simulink model "SwitchActionSubsystem"  (R2021a)
settings: Solver=VariableStepAuto  StartTime=0.0  StopTime=10.0  RelTol=1e-3
settings Model: Creator=lenovo  LastModifiedBy=lenovo

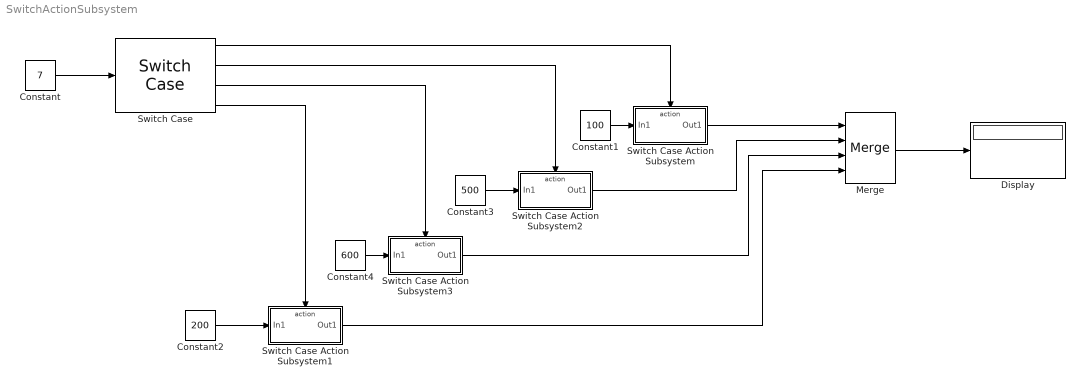
== system SwitchActionSubsystem ==
  Constant : Constant  Value=7
  Constant1 : Constant  Value=100
  Constant2 : Constant  Value=200
  Constant3 : Constant  Value=500
  Constant4 : Constant  Value=600
  Display : Display
  Merge : Merge  Inputs=4
  Switch Case : SwitchCase  CaseConditions={1,2,[4 5]}
  Switch Case Action Subsystem : Subsystem  TreatAsAtomicUnit=on
  Switch Case Action Subsystem1 : Subsystem  TreatAsAtomicUnit=on
  Switch Case Action Subsystem2 : Subsystem  TreatAsAtomicUnit=on
  Switch Case Action Subsystem3 : Subsystem  TreatAsAtomicUnit=on
  wires:
  Constant/1 -> Switch Case/1
  Switch Case/1 -> Switch Case Action Subsystem/Action
  Constant1/1 -> Switch Case Action Subsystem/1(In1)
  Constant2/1 -> Switch Case Action Subsystem1/1(In1)
  Constant3/1 -> Switch Case Action Subsystem2/1(In1)
  Switch Case/2 -> Switch Case Action Subsystem2/Action
  Switch Case/3 -> Switch Case Action Subsystem3/Action
  Constant4/1 -> Switch Case Action Subsystem3/1(In1)
  Switch Case/4 -> Switch Case Action Subsystem1/Action
  Switch Case Action Subsystem/1(Out1) -> Merge/1
  Switch Case Action Subsystem2/1(Out1) -> Merge/2
  Switch Case Action Subsystem3/1(Out1) -> Merge/3
  Switch Case Action Subsystem1/1(Out1) -> Merge/4
  Merge/1 -> Display/1

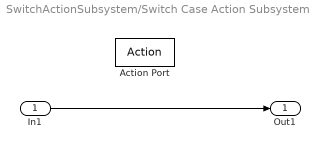
== system SwitchActionSubsystem/Switch Case Action Subsystem ==
  In1 : Inport
  Action Port : ActionPort  ActionPortLabel=case [ 1 ]:
  Out1 : Outport
  wires:
  In1/1 -> Out1/1

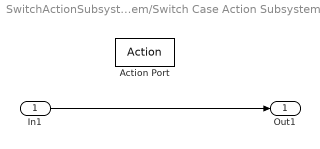
== system SwitchActionSubsystem/Switch Case Action Subsystem1 ==
  In1 : Inport
  Action Port : ActionPort  ActionPortLabel=default:
  Out1 : Outport
  wires:
  In1/1 -> Out1/1

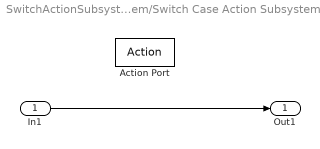
== system SwitchActionSubsystem/Switch Case Action Subsystem2 ==
  In1 : Inport
  Action Port : ActionPort  ActionPortLabel=case [ 2 ]:
  Out1 : Outport
  wires:
  In1/1 -> Out1/1

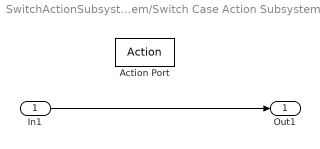
== system SwitchActionSubsystem/Switch Case Action Subsystem3 ==
  In1 : Inport
  Action Port : ActionPort  ActionPortLabel=case [ 4 5 ]:
  Out1 : Outport
  wires:
  In1/1 -> Out1/1
